simulink model "aufgabe_b2"  (R2016b)
settings: Solver=VariableStepAuto  StartTime=0.0  StopTime=10.0  RelTol=1e-3
settings Model: Creator=Thomas  LastModifiedBy=Thomas

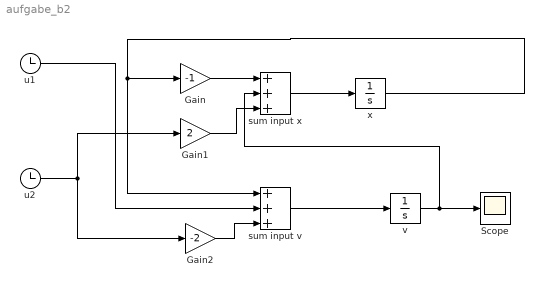
== system aufgabe_b2 ==
  Gain : Gain  Gain=-1
  Gain1 : Gain  Gain=2
  Gain2 : Gain  Gain=-2
  Scope : Scope
  sum input v : Sum  Inputs=+++
  sum input x : Sum  Inputs=+++
  u1 : Clock
  u2 : Clock
  v : Integrator
  x : Integrator
  wires:
  x/1 -> Gain/1, sum input v/1
  sum input x/1 -> x/1
  v/1 -> Scope/1, sum input x/2
  sum input v/1 -> v/1
  u2/1 -> Gain2/1, Gain1/1
  u1/1 -> sum input v/2
  Gain/1 -> sum input x/1
  Gain1/1 -> sum input x/3
  Gain2/1 -> sum input v/3
